simulink model "test_HDS_Room"  (R2019b)
settings: Solver=VariableStepAuto  StartTime=0.0  StopTime=60  MaxStep=0.01  RelTol=1e-3
undefined symbols (not defined in the file): Rec, SDTV
libraries: simulink x4, visionconversions x1, vrlib x1
settings Model: EnablePacing=on  Creator=michi  LastModifiedBy=toons
settings DataIOCC: ReturnWorkspaceOutputs=off
settings DebuggingCC: ArithmeticOperatorsInVariantConditions=warning
settings SFSimCC: CustomCodeUndefinedFunction=UseInterfaceOnly

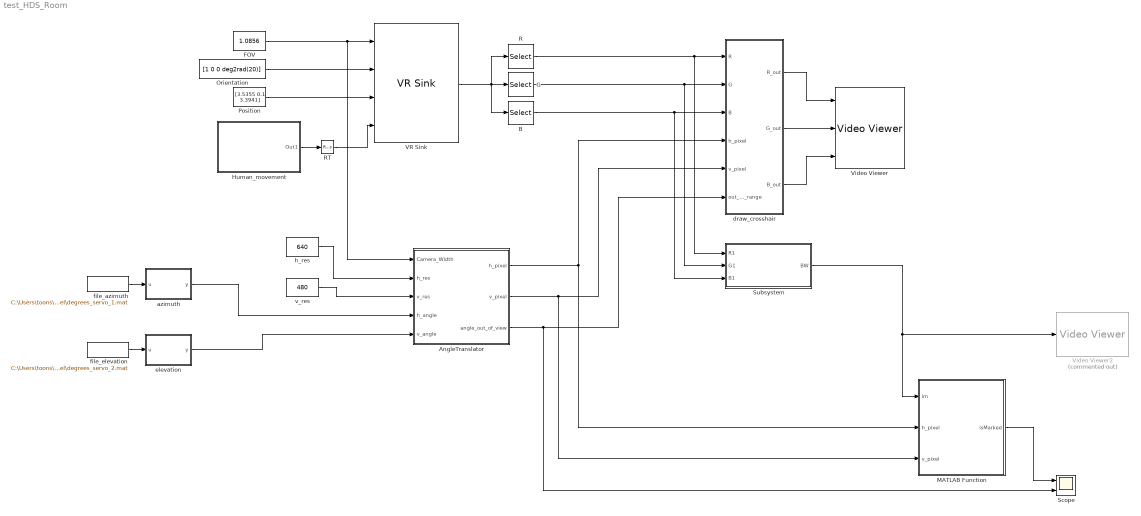
== system test_HDS_Room ==
  AngleTranslator : Subsystem
  B : Selector  NumberOfDimensions=3  InputPortWidth=3  IndexOptions=Select all,Select all,Index vector (dialog)  Indices=[1 3],1,3  OutputSizes=1,1,1
  FOV : Constant  Value=1.0856
  G : Selector  NumberOfDimensions=3  InputPortWidth=3  IndexOptions=Select all,Select all,Index vector (dialog)  Indices=[1 3],1,2  OutputSizes=1,1,1
  "Human_movement " : Subsystem
  MATLAB Function : MATLAB Function  TreatAsAtomicUnit=on
  Orientation : Constant  Value=[1 0 0 deg2rad(20)]
  Position : Constant  Value=[3.5355 0.1 3.3941]
  R : Selector  NumberOfDimensions=3  InputPortWidth=3  IndexOptions=Select all,Select all,Index vector (dialog)  Indices=[1 3],1,1  OutputSizes=1,1,1
  RT : RateTransition  OutPortSampleTime=0.1
  Scope : Scope  NumInputPorts=2
  Subsystem : Subsystem
  VR Sink : vrlib/VR Sink  InstantiateOnLoad=on  SampleTime=0.1  ViewEnable=on  RemoteChange=off  RemoteView=off  FieldsWritten=Camera.fieldOfView.1.1.1.double#Camera.orientation.4.1.1.double#Camera.position.3.1.1.double#Human.translation.3.1.1.double  WorldFileName=HDS_Room_rotated.wrl  AutoView=off  VideoDimensions=[480 640]  AllowVariableSize=off
      settings: SourceProductBaseCode=VR
  Video Viewer : VideoViewer  imagePorts=separate color signals  FigPos=[-959 1038 960 938]
  Video Viewer2 : VideoViewer  Commented=on  FigPos=[-1919 1038 1920 938]
  azimuth : MATLAB Function  TreatAsAtomicUnit=on
  draw_crosshair : Subsystem
  elevation : MATLAB Function  TreatAsAtomicUnit=on
  file_azimuth : FromFile  FileName=C:\Users\toons\Documents\MATLAB\II-CPS\Matlab\Simulink_Model\degrees_servo_1.mat  SampleTime=0
  file_elevation : FromFile  FileName=C:\Users\toons\Documents\MATLAB\II-CPS\Matlab\Simulink_Model\degrees_servo_2.mat  SampleTime=0
  h_res : Constant  Value=640
  v_res : Constant  Value=480
  wires:
  "Human_movement "/1(Out1) -> RT/1
  RT/1 -> VR Sink/4
  FOV/1 -> AngleTranslator/1(Camera_Width), VR Sink/1
  Orientation/1 -> VR Sink/2
  Position/1 -> VR Sink/3
  draw_crosshair/3(B_out) -> Video Viewer/3
  AngleTranslator/3(angle_out_of_view) -> draw_crosshair/6(out_of_range), Scope/2
  draw_crosshair/2(G_out) -> Video Viewer/2
  G/1 -> draw_crosshair/2(G), Subsystem/2(G1)
  Subsystem/1(BW) -> MATLAB Function/1(im), Video Viewer2/1
  draw_crosshair/1(R_out) -> Video Viewer/1
  AngleTranslator/1(h_pixel) -> draw_crosshair/4(h_pixel), MATLAB Function/2(h_pixel)
  AngleTranslator/2(v_pixel) -> draw_crosshair/5(v_pixel), MATLAB Function/3(v_pixel)
  MATLAB Function/1(isMarked) -> Scope/1
  VR Sink/1 -> B/1, R/1, G/1
  B/1 -> draw_crosshair/3(B), Subsystem/3(B1)
  R/1 -> draw_crosshair/1(R), Subsystem/1(R1)
  v_res/1 -> AngleTranslator/3(v_res)
  h_res/1 -> AngleTranslator/2(h_res)
  azimuth/1(y) -> AngleTranslator/4(h_angle)
  file_elevation/1 -> elevation/1(u)
  file_azimuth/1 -> azimuth/1(u)
  elevation/1(y) -> AngleTranslator/5(v_angle)

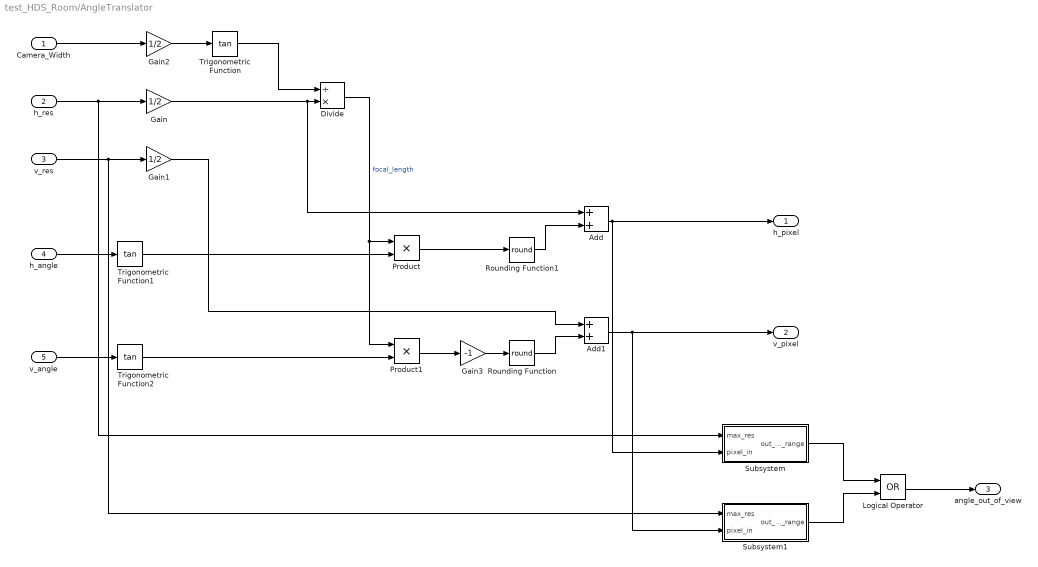
== system test_HDS_Room/AngleTranslator ==
  Camera_Width : Inport
  h_res : Inport  Port=2
  v_res : Inport  Port=3
  h_angle : Inport  Port=4
  v_angle : Inport  Port=5
  Add : Sum
  Add1 : Sum
  Divide : Product  Inputs=/*
  Gain : Gain  Gain=1/2
  Gain1 : Gain  Gain=1/2
  Gain2 : Gain  Gain=1/2
  Gain3 : Gain  Gain=-1
  Logical Operator : Logic  Operator=OR  AllPortsSameDT=off  OutDataTypeStr=boolean
  Product : Product
  Product1 : Product
  Rounding Function : Rounding  Operator=round
  Rounding Function1 : Rounding  Operator=round
  Subsystem : Subsystem
  Subsystem1 : Subsystem
  Trigonometric Function : Trigonometry  Operator=tan
  Trigonometric Function1 : Trigonometry  Operator=tan
  Trigonometric Function2 : Trigonometry  Operator=tan
  h_pixel : Outport
  v_pixel : Outport  Port=2
  angle_out_of_view : Outport  Port=3
  wires:
  h_res/1 -> Gain/1, Subsystem/1(max_res)
  v_res/1 -> Gain1/1, Subsystem1/1(max_res)
  Camera_Width/1 -> Gain2/1
  Gain2/1 -> Trigonometric Function/1
  h_angle/1 -> Trigonometric Function1/1
  v_angle/1 -> Trigonometric Function2/1
  Trigonometric Function1/1 -> Product/2
  Divide/1 -> Product/1, Product1/1  "focal_length"
  Trigonometric Function2/1 -> Product1/2
  Gain/1 -> Add/1, Divide/2
  Trigonometric Function/1 -> Divide/1
  Product1/1 -> Gain3/1
  Product/1 -> Rounding Function1/1
  Gain3/1 -> Rounding Function/1
  Rounding Function1/1 -> Add/2
  Rounding Function/1 -> Add1/2
  Gain1/1 -> Add1/1
  Add1/1 -> Subsystem1/2(pixel_in), v_pixel/1
  Add/1 -> Subsystem/2(pixel_in), h_pixel/1
  Logical Operator/1 -> angle_out_of_view/1
  Subsystem/1(out_of_range) -> Logical Operator/1
  Subsystem1/1(out_of_range) -> Logical Operator/2

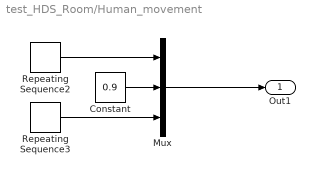
== system test_HDS_Room/Human_movement  ==
  Constant : Constant  Value=0.9
  Mux : Mux  Inputs=3
  Repeating Sequence2 : simulink/Sources/Repeating Sequence  rep_seq_t=[0 3 4 7 8 11 12 15 16]  rep_seq_y=[1 3.5 3.5 6 6 3.5 3.5 1 1]
  Repeating Sequence3 : simulink/Sources/Repeating Sequence  rep_seq_t=[0 3 4 7 8 11 12 15 16]  rep_seq_y=[0 -2.5 -2.5 0 0 2.5 2.5 0 0]
  Out1 : Outport  VectorParamsAs1DForOutWhenUnconnected=off
  wires:
  Mux/1 -> Out1/1
  Constant/1 -> Mux/2
  Repeating Sequence2/1 -> Mux/1
  Repeating Sequence3/1 -> Mux/3

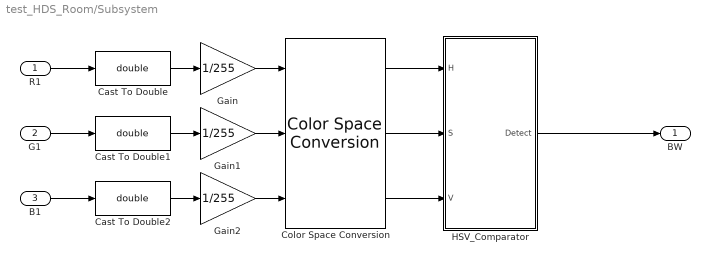
== system test_HDS_Room/Subsystem ==
  R1 : Inport
  G1 : Inport  Port=2
  B1 : Inport  Port=3
  Cast To Double : DataTypeConversion  OutDataTypeStr=double
  Cast To Double1 : DataTypeConversion  OutDataTypeStr=double
  Cast To Double2 : DataTypeConversion  OutDataTypeStr=double
  Color Space Conversion : visionconversions/Color Space  Conversion  conversion=Obsolete  conversionActive=R'G'B' to HSV  wp_str=D65  rec=Rec. 601 (SDTV)  sys=1125/60/2:1  imagePorts=Separate color signals
  Gain : Gain  Gain=1/255
  Gain1 : Gain  Gain=1/255
  Gain2 : Gain  Gain=1/255
  HSV_Comparator : Subsystem
  BW : Outport
  wires:
  Cast To Double/1 -> Gain/1
  Gain2/1 -> Color Space Conversion/3
  Cast To Double2/1 -> Gain2/1
  G1/1 -> Cast To Double1/1
  Color Space Conversion/1 -> HSV_Comparator/1(H)
  Color Space Conversion/3 -> HSV_Comparator/3(V)
  B1/1 -> Cast To Double2/1
  Cast To Double1/1 -> Gain1/1
  Gain/1 -> Color Space Conversion/1
  R1/1 -> Cast To Double/1
  HSV_Comparator/1(Detect) -> BW/1
  Gain1/1 -> Color Space Conversion/2
  Color Space Conversion/2 -> HSV_Comparator/2(S)

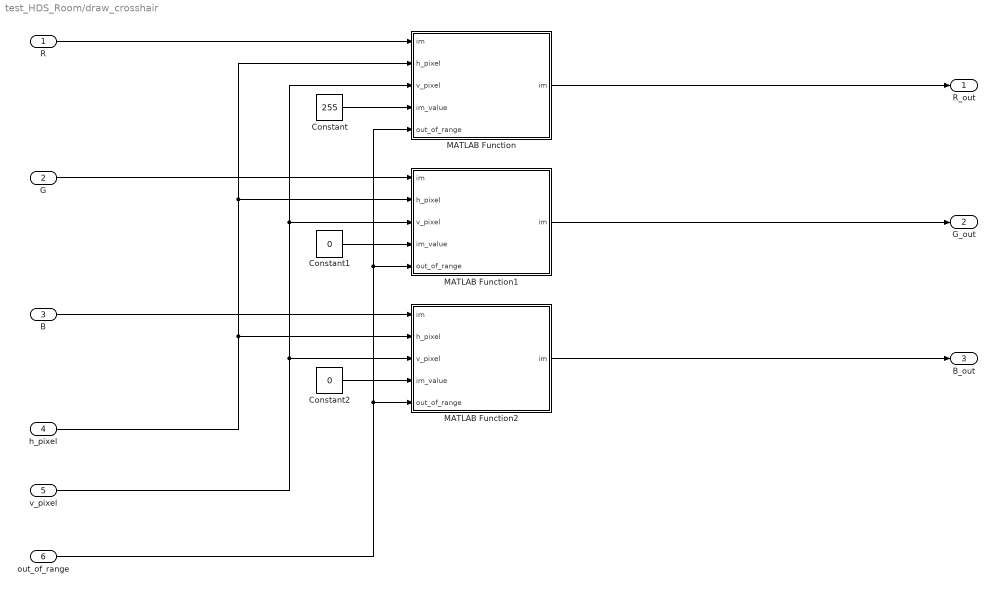
== system test_HDS_Room/draw_crosshair ==
  R : Inport
  G : Inport  Port=2
  B : Inport  Port=3
  h_pixel : Inport  Port=4
  v_pixel : Inport  Port=5
  out_of_range : Inport  Port=6
  Constant : Constant  Value=255
  Constant1 : Constant  Value=0
  Constant2 : Constant  Value=0
  MATLAB Function : MATLAB Function  TreatAsAtomicUnit=on
  MATLAB Function1 : MATLAB Function  TreatAsAtomicUnit=on
  MATLAB Function2 : MATLAB Function  TreatAsAtomicUnit=on
  R_out : Outport
  G_out : Outport  Port=2
  B_out : Outport  Port=3
  wires:
  R/1 -> MATLAB Function/1("im ")
  h_pixel/1 -> MATLAB Function2/2(h_pixel), MATLAB Function/2(h_pixel), MATLAB Function1/2(h_pixel)
  v_pixel/1 -> MATLAB Function2/3(v_pixel), MATLAB Function1/3(v_pixel), MATLAB Function/3(v_pixel)
  out_of_range/1 -> MATLAB Function2/5(out_of_range), MATLAB Function1/5(out_of_range), MATLAB Function/5(out_of_range)
  Constant/1 -> MATLAB Function/4(im_value)
  MATLAB Function/1(im) -> R_out/1
  G/1 -> MATLAB Function1/1("im ")
  B/1 -> MATLAB Function2/1("im ")
  Constant1/1 -> MATLAB Function1/4(im_value)
  Constant2/1 -> MATLAB Function2/4(im_value)
  MATLAB Function2/1(im) -> B_out/1
  MATLAB Function1/1(im) -> G_out/1

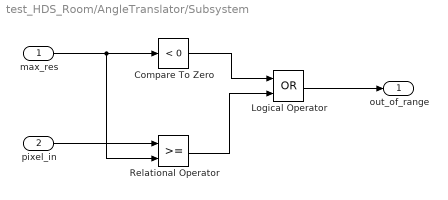
== system test_HDS_Room/AngleTranslator/Subsystem ==
  max_res : Inport
  pixel_in : Inport  Port=2
  Compare To Zero : simulink/Logic and Bit Operations/Compare To Zero  relop=<  OutDataTypeStr=boolean
  Logical Operator : Logic  Operator=OR  AllPortsSameDT=off  OutDataTypeStr=boolean
  Relational Operator : RelationalOperator  OutDataTypeStr=boolean  RndMeth=Simplest
  out_of_range : Outport
  wires:
  pixel_in/1 -> Relational Operator/1
  max_res/1 -> Compare To Zero/1, Relational Operator/2
  Logical Operator/1 -> out_of_range/1
  Compare To Zero/1 -> Logical Operator/1
  Relational Operator/1 -> Logical Operator/2

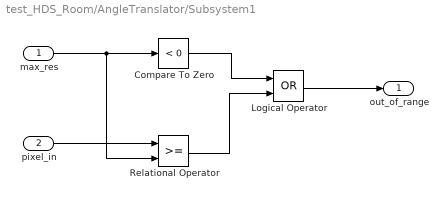
== system test_HDS_Room/AngleTranslator/Subsystem1 ==
  max_res : Inport
  pixel_in : Inport  Port=2
  Compare To Zero : simulink/Logic and Bit Operations/Compare To Zero  relop=<  OutDataTypeStr=boolean
  Logical Operator : Logic  Operator=OR  AllPortsSameDT=off  OutDataTypeStr=boolean
  Relational Operator : RelationalOperator  OutDataTypeStr=boolean  RndMeth=Simplest
  out_of_range : Outport
  wires:
  pixel_in/1 -> Relational Operator/1
  max_res/1 -> Compare To Zero/1, Relational Operator/2
  Logical Operator/1 -> out_of_range/1
  Compare To Zero/1 -> Logical Operator/1
  Relational Operator/1 -> Logical Operator/2

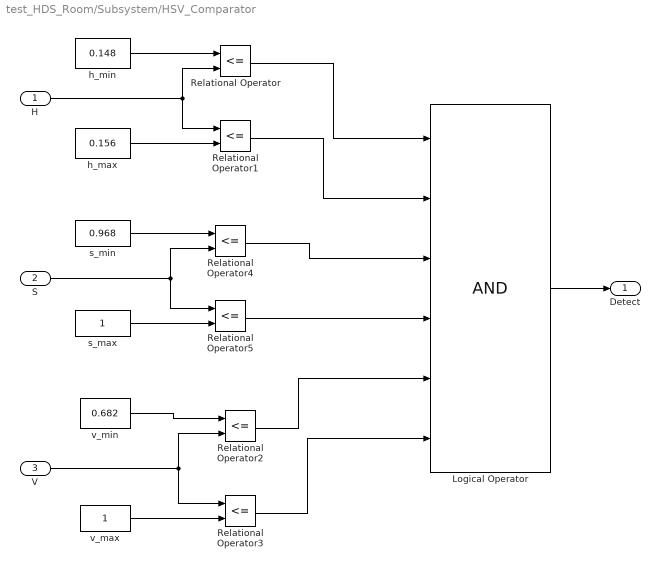
== system test_HDS_Room/Subsystem/HSV_Comparator ==
  H : Inport
  S : Inport  Port=2
  V : Inport  Port=3
  Logical Operator : Logic  Inputs=6  AllPortsSameDT=off  OutDataTypeStr=boolean
  Relational Operator{,1..5} (6 alike) : RelationalOperator  Operator=<=  OutDataTypeStr=boolean  RndMeth=Simplest
  h_max : Constant  Value=0.156
  h_min : Constant  Value=0.148
  s_max : Constant
  s_min : Constant  Value=0.968
  v_max : Constant
  v_min : Constant  Value=0.682
  Detect : Outport
  wires:
  h_min/1 -> Relational Operator/1
  H/1 -> Relational Operator1/1, Relational Operator/2
  h_max/1 -> Relational Operator1/2
  s_min/1 -> Relational Operator4/1
  S/1 -> Relational Operator5/1, Relational Operator4/2
  s_max/1 -> Relational Operator5/2
  v_min/1 -> Relational Operator2/1
  V/1 -> Relational Operator3/1, Relational Operator2/2
  v_max/1 -> Relational Operator3/2
  Relational Operator/1 -> Logical Operator/1
  Relational Operator1/1 -> Logical Operator/2
  Relational Operator4/1 -> Logical Operator/3
  Relational Operator5/1 -> Logical Operator/4
  Relational Operator2/1 -> Logical Operator/5
  Relational Operator3/1 -> Logical Operator/6
  Logical Operator/1 -> Detect/1

== matlab function test_HDS_Room/draw_crosshair/MATLAB Function ==
  data: im input; im output; h_pixel input; v_pixel input; im_value input; out_of_range input
function im = draw_crosshair(im, h_pixel, v_pixel, im_value, out_of_range)

h_pixel = max(1, h_pixel);
v_pixel = max(1, v_pixel);

h_max = size(im, 2);
v_max = size(im, 1);

h_pixel = min(h_max, h_pixel);
v_pixel = min(v_max, v_pixel);

if out_of_range == 0
    im(:,h_pixel) = im_value;
    im(v_pixel,:) = im_value;
end

== matlab function test_HDS_Room/MATLAB Function ==
  data: im input; isMarked output; h_pixel input; v_pixel input
function isMarked  = PixelCompare(im, h_pixel, v_pixel)
%PIXELCOMPARE Check if a pixel is marked
%   This function checks a BW image to see if the pixel is marked. It
%   returns 1 if the pixel is marked, 0 if the pixel is unmarked.
h_pixel = max(1, h_pixel);
v_pixel = max(1, v_pixel);

h_max = size(im, 2);
v_max = size(im, 1);

h_pixel = min(h_max, h_pixel);
v_pixel = min(v_max, v_pixel);

isMarked = im(v_pixel,h_pixel);
end

== matlab function test_HDS_Room/draw_crosshair/MATLAB Function1 ==
  data: im input; im output; h_pixel input; v_pixel input; im_value input; out_of_range input
function im = draw_crosshair(im, h_pixel, v_pixel, im_value, out_of_range)

h_pixel = max(1, h_pixel);
v_pixel = max(1, v_pixel);

h_max = size(im, 2);
v_max = size(im, 1);

h_pixel = min(h_max, h_pixel);
v_pixel = min(v_max, v_pixel);

if out_of_range == 0
    im(:,h_pixel) = im_value;
    im(v_pixel,:) = im_value;
end

== matlab function test_HDS_Room/draw_crosshair/MATLAB Function2 ==
  data: im input; im output; h_pixel input; v_pixel input; im_value input; out_of_range input
function im = draw_crosshair(im, h_pixel, v_pixel, im_value, out_of_range)

h_pixel = max(1, h_pixel);
v_pixel = max(1, v_pixel);

h_max = size(im, 2);
v_max = size(im, 1);

h_pixel = min(h_max, h_pixel);
v_pixel = min(v_max, v_pixel);

if out_of_range == 0
    im(:,h_pixel) = im_value;
    im(v_pixel,:) = im_value;
end

== matlab function test_HDS_Room/azimuth ==
  data: u input; y output
function y = fcn(u)
y = ((-1)*u)+90 - 45;
y = deg2rad(y);

== matlab function test_HDS_Room/elevation ==
  data: u input; y output
function y = fcn(u)
u = u*(-1);
y = u + 90 -20;
y = deg2rad(y);
